simulink library "GFo_Lib"  (R2020b)
settings: Solver=VariableStepAuto  StartTime=0.0  StopTime=10.0  RelTol=1e-3
values from neighbouring files (symbols this model uses):
  Cb = 1/(Zb*wb)    [Init_Base_SM.m]
  fb = fn    [Init_Base_SM.m]
  Ib1 = Sb / (3*Vb1)    [Init_Base_SM.m]
  Ib2 = Sb / (3*Vb2)    [Init_Base_SM.m]
  Lb = Zb/wb    [Init_Base_SM.m]
  Sb = Pb/cos_phi_n    [Init_Base_SM.m]
  Va0 = Vvsc0*sqrt(2)*Vb1*sin(Theta_vsc0*pi/180)    [Init_LF_L_mod.m]
  Vb0 = Vvsc0*sqrt(2)*Vb1*sin(Theta_vsc0*pi/180-2*pi/3)    [Init_LF_L_mod.m]
  Vb1 = Vn1    [Init_Base_SM.m]
  Vb2 = Vn2    [Init_Base_SM.m]
  Vc0 = Vvsc0*sqrt(2)*Vb1*sin(Theta_vsc0*pi/180+2*pi/3)    [Init_LF_L_mod.m]
  Vvsc0 = abs(V1)    [Init_LF_L_mod.m]    (also in Init_LF_SM.m = Vm0)
  Zb = (3*Vb1^2)/Sb    [Init_Base_SM.m]
undefined symbols (not defined in the file or in its folder): C_line, DiscIntNeverNeededParam, Eg0, Is0_d, Is0_q, Kp_Rvi_pu, Time_Step, Ug, VSC01_id0
libraries: powerlib x152, Control_Lib x35, powerlib_meascontrol x10, simulink x6
(part 5 of 5)

== system GFo_Lib/MMC_GFM_EB/Bridge_Model/MMC Average Model/Arm_la ==
  m : Inport
  Controlled Current Source : powerlib/Electrical Sources/Controlled Current Source  Initialize=on  Source_Type=DC  Amplitude=0  Phase=0  Frequency=0  Measurements=None
  Controlled Voltage Source2 : powerlib/Electrical Sources/Controlled Voltage Source  Initialize=on  Source_Type=DC  Amplitude=Vdc/2  Phase=180  Frequency=0  Measurements=None
  Current Measurement7 : powerlib/Measurements/Current Measurement  PhasorSimulation=off  OutputType=Complex  PSBequivalent=0
  Memory1 : Memory  InitialCondition=Vdc/2
  Memory2 : Memory
  Product : Product  RndMeth=Zero
  Product1 : Product  RndMeth=Zero
  Series RLC Branch : powerlib/Elements/Series RLC Branch  LConnTagsString=__new0  RConnTagsString=__new0  BranchType=C  Resistance=1  Inductance=1e-3  SetiL0=off  InitialCurrent=0  Capacitance=C_arm  Setx0=on  InitialVoltage=Vdc  Measurements=None
  Voltage Measurement : powerlib/Measurements/Voltage Measurement  PhasorSimulation=off  OutputType=Complex  PSBequivalent=0
  Voltage Measurement1 : powerlib/Measurements/Voltage Measurement  PhasorSimulation=off  OutputType=Complex  PSBequivalent=0
  V+ : PMIOPort  Side=Left
  V- : PMIOPort  Port=2  Side=Left
  vctot : Outport
  i_arm : Outport  Port=2
  v_arm : Outport  Port=3
  wires:
  Memory1/1 -> Controlled Voltage Source2/1
  Memory2/1 -> Controlled Current Source/1
  Product/1 -> Memory1/1
  Voltage Measurement/1 -> v_arm/1
  Product1/1 -> Memory2/1
  m/1 -> [m], Product1/1
  Current Measurement7/1 -> i_arm/1, Product1/2
  [m] -> Product/2
  Voltage Measurement1/1 -> Product/1, vctot/1
  connections:
  Current Measurement7/RConn1 -- Controlled Voltage Source2/RConn1
  Current Measurement7/LConn1 -- Voltage Measurement/LConn1 -- V+/RConn1
  Controlled Current Source/LConn1 -- Series RLC Branch/RConn1 -- Voltage Measurement1/LConn2 -- V-/RConn1 -- Voltage Measurement/LConn2 -- Controlled Voltage Source2/LConn1
  Controlled Current Source/RConn1 -- Series RLC Branch/LConn1 -- Voltage Measurement1/LConn1

== system GFo_Lib/MMC_GFM_EB/Bridge_Model/MMC Average Model/Arm_lb ==
  m : Inport
  Controlled Current Source : powerlib/Electrical Sources/Controlled Current Source  Initialize=on  Source_Type=DC  Amplitude=0  Phase=0  Frequency=0  Measurements=None
  Controlled Voltage Source2 : powerlib/Electrical Sources/Controlled Voltage Source  Initialize=on  Source_Type=DC  Amplitude=Vdc/2  Phase=180  Frequency=0  Measurements=None
  Current Measurement7 : powerlib/Measurements/Current Measurement  PhasorSimulation=off  OutputType=Complex  PSBequivalent=0
  Memory1 : Memory  InitialCondition=Vdc/2
  Memory2 : Memory
  Product : Product  RndMeth=Zero
  Product1 : Product  RndMeth=Zero
  Series RLC Branch : powerlib/Elements/Series RLC Branch  LConnTagsString=__new0  RConnTagsString=__new0  BranchType=C  Resistance=1  Inductance=1e-3  SetiL0=off  InitialCurrent=0  Capacitance=C_arm  Setx0=on  InitialVoltage=Vdc  Measurements=None
  Voltage Measurement : powerlib/Measurements/Voltage Measurement  PhasorSimulation=off  OutputType=Complex  PSBequivalent=0
  Voltage Measurement1 : powerlib/Measurements/Voltage Measurement  PhasorSimulation=off  OutputType=Complex  PSBequivalent=0
  V+ : PMIOPort  Side=Left
  V- : PMIOPort  Port=2  Side=Left
  vctot : Outport
  i_arm : Outport  Port=2
  v_arm : Outport  Port=3
  wires:
  Memory1/1 -> Controlled Voltage Source2/1
  Memory2/1 -> Controlled Current Source/1
  Product/1 -> Memory1/1
  Voltage Measurement/1 -> v_arm/1
  Product1/1 -> Memory2/1
  m/1 -> [m], Product1/1
  Current Measurement7/1 -> i_arm/1, Product1/2
  [m] -> Product/2
  Voltage Measurement1/1 -> Product/1, vctot/1
  connections:
  Current Measurement7/RConn1 -- Controlled Voltage Source2/RConn1
  Current Measurement7/LConn1 -- Voltage Measurement/LConn1 -- V+/RConn1
  Controlled Current Source/LConn1 -- Series RLC Branch/RConn1 -- Voltage Measurement1/LConn2 -- V-/RConn1 -- Voltage Measurement/LConn2 -- Controlled Voltage Source2/LConn1
  Controlled Current Source/RConn1 -- Series RLC Branch/LConn1 -- Voltage Measurement1/LConn1

== system GFo_Lib/MMC_GFM_EB/Bridge_Model/MMC Average Model/Arm_lc ==
  m : Inport
  Controlled Current Source : powerlib/Electrical Sources/Controlled Current Source  Initialize=on  Source_Type=DC  Amplitude=0  Phase=0  Frequency=0  Measurements=None
  Controlled Voltage Source2 : powerlib/Electrical Sources/Controlled Voltage Source  Initialize=on  Source_Type=DC  Amplitude=Vdc/2  Phase=180  Frequency=0  Measurements=None
  Current Measurement7 : powerlib/Measurements/Current Measurement  PhasorSimulation=off  OutputType=Complex  PSBequivalent=0
  Memory1 : Memory  InitialCondition=Vdc/2
  Memory2 : Memory
  Product : Product  RndMeth=Zero
  Product1 : Product  RndMeth=Zero
  Series RLC Branch : powerlib/Elements/Series RLC Branch  LConnTagsString=__new0  RConnTagsString=__new0  BranchType=C  Resistance=1  Inductance=1e-3  SetiL0=off  InitialCurrent=0  Capacitance=C_arm  Setx0=on  InitialVoltage=Vdc  Measurements=None
  Voltage Measurement : powerlib/Measurements/Voltage Measurement  PhasorSimulation=off  OutputType=Complex  PSBequivalent=0
  Voltage Measurement1 : powerlib/Measurements/Voltage Measurement  PhasorSimulation=off  OutputType=Complex  PSBequivalent=0
  V+ : PMIOPort  Side=Left
  V- : PMIOPort  Port=2  Side=Left
  vctot : Outport
  i_arm : Outport  Port=2
  v_arm : Outport  Port=3
  wires:
  Memory1/1 -> Controlled Voltage Source2/1
  Memory2/1 -> Controlled Current Source/1
  Product/1 -> Memory1/1
  Voltage Measurement/1 -> v_arm/1
  Product1/1 -> Memory2/1
  m/1 -> [m], Product1/1
  Current Measurement7/1 -> i_arm/1, Product1/2
  [m] -> Product/2
  Voltage Measurement1/1 -> Product/1, vctot/1
  connections:
  Current Measurement7/RConn1 -- Controlled Voltage Source2/RConn1
  Current Measurement7/LConn1 -- Voltage Measurement/LConn1 -- V+/RConn1
  Controlled Current Source/LConn1 -- Series RLC Branch/RConn1 -- Voltage Measurement1/LConn2 -- V-/RConn1 -- Voltage Measurement/LConn2 -- Controlled Voltage Source2/LConn1
  Controlled Current Source/RConn1 -- Series RLC Branch/LConn1 -- Voltage Measurement1/LConn1

== system GFo_Lib/MMC_GFM_EB/Bridge_Model/MMC Average Model/Arm_ua ==
  m : Inport
  Controlled Current Source : powerlib/Electrical Sources/Controlled Current Source  Initialize=on  Source_Type=DC  Amplitude=0  Phase=0  Frequency=0  Measurements=None
  Controlled Voltage Source2 : powerlib/Electrical Sources/Controlled Voltage Source  Initialize=on  Source_Type=DC  Amplitude=Vdc/2  Phase=180  Frequency=0  Measurements=None
  Current Measurement7 : powerlib/Measurements/Current Measurement  PhasorSimulation=off  OutputType=Complex  PSBequivalent=0
  Memory1 : Memory  InitialCondition=Vdc/2
  Memory2 : Memory
  Product : Product  RndMeth=Zero
  Product1 : Product  RndMeth=Zero
  Series RLC Branch : powerlib/Elements/Series RLC Branch  LConnTagsString=__new0  RConnTagsString=__new0  BranchType=C  Resistance=1  Inductance=1e-3  SetiL0=off  InitialCurrent=0  Capacitance=C_arm  Setx0=on  InitialVoltage=Vdc  Measurements=None
  Voltage Measurement : powerlib/Measurements/Voltage Measurement  PhasorSimulation=off  OutputType=Complex  PSBequivalent=0
  Voltage Measurement1 : powerlib/Measurements/Voltage Measurement  PhasorSimulation=off  OutputType=Complex  PSBequivalent=0
  V+ : PMIOPort  Side=Left
  V- : PMIOPort  Port=2  Side=Left
  vctot : Outport
  i_arm : Outport  Port=2
  v_arm : Outport  Port=3
  wires:
  Memory1/1 -> Controlled Voltage Source2/1
  Memory2/1 -> Controlled Current Source/1
  Product/1 -> Memory1/1
  Voltage Measurement/1 -> v_arm/1
  Product1/1 -> Memory2/1
  m/1 -> [m], Product1/1
  Current Measurement7/1 -> i_arm/1, Product1/2
  [m] -> Product/2
  Voltage Measurement1/1 -> Product/1, vctot/1
  connections:
  Current Measurement7/RConn1 -- Controlled Voltage Source2/RConn1
  Current Measurement7/LConn1 -- Voltage Measurement/LConn1 -- V+/RConn1
  Controlled Current Source/LConn1 -- Series RLC Branch/RConn1 -- Voltage Measurement1/LConn2 -- V-/RConn1 -- Voltage Measurement/LConn2 -- Controlled Voltage Source2/LConn1
  Controlled Current Source/RConn1 -- Series RLC Branch/LConn1 -- Voltage Measurement1/LConn1

== system GFo_Lib/MMC_GFM_EB/Bridge_Model/MMC Average Model/Arm_ub ==
  m : Inport
  Controlled Current Source : powerlib/Electrical Sources/Controlled Current Source  Initialize=on  Source_Type=DC  Amplitude=0  Phase=0  Frequency=0  Measurements=None
  Controlled Voltage Source2 : powerlib/Electrical Sources/Controlled Voltage Source  Initialize=on  Source_Type=DC  Amplitude=Vdc/2  Phase=180  Frequency=0  Measurements=None
  Current Measurement7 : powerlib/Measurements/Current Measurement  PhasorSimulation=off  OutputType=Complex  PSBequivalent=0
  Memory1 : Memory  InitialCondition=Vdc/2
  Memory2 : Memory
  Product : Product  RndMeth=Zero
  Product1 : Product  RndMeth=Zero
  Series RLC Branch : powerlib/Elements/Series RLC Branch  LConnTagsString=__new0  RConnTagsString=__new0  BranchType=C  Resistance=1  Inductance=1e-3  SetiL0=off  InitialCurrent=0  Capacitance=C_arm  Setx0=on  InitialVoltage=Vdc  Measurements=None
  Voltage Measurement : powerlib/Measurements/Voltage Measurement  PhasorSimulation=off  OutputType=Complex  PSBequivalent=0
  Voltage Measurement1 : powerlib/Measurements/Voltage Measurement  PhasorSimulation=off  OutputType=Complex  PSBequivalent=0
  V+ : PMIOPort  Side=Left
  V- : PMIOPort  Port=2  Side=Left
  vctot : Outport
  i_arm : Outport  Port=2
  v_arm : Outport  Port=3
  wires:
  Memory1/1 -> Controlled Voltage Source2/1
  Memory2/1 -> Controlled Current Source/1
  Product/1 -> Memory1/1
  Voltage Measurement/1 -> v_arm/1
  Product1/1 -> Memory2/1
  m/1 -> [m], Product1/1
  Current Measurement7/1 -> i_arm/1, Product1/2
  [m] -> Product/2
  Voltage Measurement1/1 -> Product/1, vctot/1
  connections:
  Current Measurement7/RConn1 -- Controlled Voltage Source2/RConn1
  Current Measurement7/LConn1 -- Voltage Measurement/LConn1 -- V+/RConn1
  Controlled Current Source/LConn1 -- Series RLC Branch/RConn1 -- Voltage Measurement1/LConn2 -- V-/RConn1 -- Voltage Measurement/LConn2 -- Controlled Voltage Source2/LConn1
  Controlled Current Source/RConn1 -- Series RLC Branch/LConn1 -- Voltage Measurement1/LConn1

== system GFo_Lib/MMC_GFM_EB/Bridge_Model/MMC Average Model/Arm_uc ==
  m : Inport
  Controlled Current Source : powerlib/Electrical Sources/Controlled Current Source  Initialize=on  Source_Type=DC  Amplitude=0  Phase=0  Frequency=0  Measurements=None
  Controlled Voltage Source2 : powerlib/Electrical Sources/Controlled Voltage Source  Initialize=on  Source_Type=DC  Amplitude=Vdc/2  Phase=180  Frequency=0  Measurements=None
  Current Measurement7 : powerlib/Measurements/Current Measurement  PhasorSimulation=off  OutputType=Complex  PSBequivalent=0
  Memory1 : Memory  InitialCondition=Vdc/2
  Memory2 : Memory
  Product : Product  RndMeth=Zero
  Product1 : Product  RndMeth=Zero
  Series RLC Branch : powerlib/Elements/Series RLC Branch  LConnTagsString=__new0  RConnTagsString=__new0  BranchType=C  Resistance=1  Inductance=1e-3  SetiL0=off  InitialCurrent=0  Capacitance=C_arm  Setx0=on  InitialVoltage=Vdc  Measurements=None
  Voltage Measurement : powerlib/Measurements/Voltage Measurement  PhasorSimulation=off  OutputType=Complex  PSBequivalent=0
  Voltage Measurement1 : powerlib/Measurements/Voltage Measurement  PhasorSimulation=off  OutputType=Complex  PSBequivalent=0
  V+ : PMIOPort  Side=Left
  V- : PMIOPort  Port=2  Side=Left
  vctot : Outport
  i_arm : Outport  Port=2
  v_arm : Outport  Port=3
  wires:
  Memory1/1 -> Controlled Voltage Source2/1
  Memory2/1 -> Controlled Current Source/1
  Product/1 -> Memory1/1
  Voltage Measurement/1 -> v_arm/1
  Product1/1 -> Memory2/1
  m/1 -> [m], Product1/1
  Current Measurement7/1 -> i_arm/1, Product1/2
  [m] -> Product/2
  Voltage Measurement1/1 -> Product/1, vctot/1
  connections:
  Current Measurement7/RConn1 -- Controlled Voltage Source2/RConn1
  Current Measurement7/LConn1 -- Voltage Measurement/LConn1 -- V+/RConn1
  Controlled Current Source/LConn1 -- Series RLC Branch/RConn1 -- Voltage Measurement1/LConn2 -- V-/RConn1 -- Voltage Measurement/LConn2 -- Controlled Voltage Source2/LConn1
  Controlled Current Source/RConn1 -- Series RLC Branch/LConn1 -- Voltage Measurement1/LConn1

== system GFo_Lib/MMC_GFM_EB/Control loops/Current Limitation/Current control ==
  Ig_dq0* : Inport
  Ig_dq0 : Inport  Port=2
  vg_dq0 : Inport  Port=3
  w : Inport  Port=4
  Demux : Demux  Outputs=2
  Demux1 : Demux  Outputs=2
  Demux2 : Demux  Outputs=2
  Gain Corrector : Gain  Gain=3/(Tr_I_max/1000)*Lt_pu
  Gain Corrector1 : Gain  Gain=3/(Tr_I_max/1000)*Lt_pu
  Mux : Mux  Inputs=2
  Product : Product  RndMeth=Zero
  Product1 : Product  RndMeth=Zero
  Sum : Sum  Inputs=|+-
  Sum2 : Sum  Inputs=|+-
  Sum3 : Sum  Inputs=|++
  Sum5 : Sum  Inputs=++|
  Sum6 : Sum  Inputs=-+|
  Sum7 : Sum  Inputs=++|
  vpcc_abc{1,3..6} (5 alike) : Scope
  w*Lf_pu : Gain  Gain=Lt_pu
  vm : Outport  InitialOutput=0  VectorParamsAs1DForOutWhenUnconnected=off
  wires:
  Demux2/2 -> Sum7/1
  Demux2/1 -> Sum3/2
  w/1 -> vpcc_abc5/1, w*Lf_pu/1
  Sum/1 -> vpcc_abc1/1, Gain Corrector/1
  Sum7/1 -> Mux/2  "Vm_q*"
  Sum3/1 -> Mux/1, vpcc_abc3/1  "Vm_d*"
  Sum5/1 -> Sum7/2
  Product1/1 -> Sum5/1
  Gain Corrector1/1 -> Sum5/2
  Demux/2 -> Sum6/2
  Sum2/1 -> Sum3/1
  Product/1 -> Sum2/2
  Demux1/2 -> Sum6/1, Product/1
  w*Lf_pu/1 -> Product/2, Product1/1
  Gain Corrector/1 -> Sum2/1
  Demux1/1 -> Sum/2, Product1/2
  Demux/1 -> Sum/1
  Ig_dq0/1 -> Demux1/1
  vg_dq0/1 -> Demux2/1, vpcc_abc6/1
  Sum6/1 -> Gain Corrector1/1
  Ig_dq0*/1 -> vpcc_abc4/1, Demux/1
  Mux/1 -> vm/1

== system GFo_Lib/MMC_GFM_EB/Control loops/Current Limitation/Inverse Current control ==
  Vm_dq* : Inport
  Ig_dq : Inport  Port=2
  vg_dq : Inport  Port=3
  w : Inport  Port=4
  Demux : Demux  Outputs=2
  Demux1 : Demux  Outputs=2
  Demux2 : Demux  Outputs=2
  Gain Corrector2 : Gain  Gain=1/(3/(Tr_I_max/1000)*Lt_pu)
  Gain Corrector3 : Gain  Gain=1/(3/(Tr_I_max/1000)*Lt_pu)
  Mux : Mux  Inputs=2
  Product : Product  RndMeth=Zero
  Product1 : Product  RndMeth=Zero
  Sum : Sum  Inputs=|+-
  Sum2 : Sum  Inputs=|++
  Sum3 : Sum  Inputs=|++
  Sum5 : Sum  Inputs=-+|
  Sum6 : Sum  Inputs=-+|
  Sum7 : Sum  Inputs=++|
  w*Lf_pu : Gain  Gain=Lt_pu
  Is_dq* : Outport  InitialOutput=0  VectorParamsAs1DForOutWhenUnconnected=off
  wires:
  vg_dq/1 -> Demux2/1
  Ig_dq/1 -> Demux1/1
  Vm_dq*/1 -> Demux/1
  Demux/1 -> Sum/1
  Demux1/1 -> Sum3/2, Product1/2
  Sum/1 -> Sum2/1
  w*Lf_pu/1 -> Product1/1, Product/2
  Product/1 -> Sum2/2
  Sum2/1 -> Gain Corrector3/1
  Mux/1 -> Is_dq*/1
  Demux/2 -> Sum6/2
  Sum6/1 -> Sum5/2
  Sum5/1 -> Gain Corrector2/1
  Sum3/1 -> Mux/1  "is_d*"
  Sum7/1 -> Mux/2  "is_q*"
  w/1 -> w*Lf_pu/1
  Demux1/2 -> Sum7/1, Product/1
  Gain Corrector3/1 -> Sum3/1
  Demux2/1 -> Sum/2
  Demux2/2 -> Sum6/1
  Product1/1 -> Sum5/1
  Gain Corrector2/1 -> Sum7/2

== system GFo_Lib/MMC_GFM_EB/Control loops/DC part: stored energy control + differential current control/Control Wdiff ==
  Wdiff pu : Inport
  Wdiff_ref pu : Inport  Port=2
  theta : Inport  Port=3
  vv_pu : Inport  Port=4
  Constant : Constant  Value=-2
  Discrete-Time Integrator : DiscreteIntegrator  SampleTime=Time_Step  ICPrevOutput=DiscIntNeverNeededParam  ICPrevScaledInput=DiscIntNeverNeededParam
  Gain5 : Gain  Gain=Vb1/Vdcb
  Gain_i 1 : Gain  Gain=Ki_Wdiff_pu  SaturateOnIntegerOverflow=on  OutDataTypeStr=Inherit: Same as input  ParamDataTypeStr=Inherit: Same as input
  Gain_i 4 : Gain  Gain=Kp_Wdiff_pu  SaturateOnIntegerOverflow=on  OutDataTypeStr=Inherit: Same as input  ParamDataTypeStr=Inherit: Same as input
  Mux1 : Mux  Inputs=3
  Mux2 : Mux  Inputs=3
  Mux3 : Mux  Inputs=3
  Mux5 : Mux  Inputs=2
  Product1 : Product  Inputs=*/*
  Sum2 : Sum  InputSameDT=on  SaturateOnIntegerOverflow=on  OutDataTypeStr=Inherit: Same as first input
  Sum3 : Sum  Inputs=+-  InputSameDT=on  SaturateOnIntegerOverflow=on  OutDataTypeStr=Inherit: Same as first input
  vsa_1 : Fcn  Expr=u(1)*cos(u(4))
  vsa_2 : Fcn  Expr=u(1)-1/2*u(2)-1/2*u(3)
  vsa_3 : Fcn  Expr=u(1)*cos(u(4))+1/3^0.5*u(2)*cos(u(4)+1/2*pi)+1/3^0.5*u(3)*cos(u(4)-1/2*pi)
  vsb_1 : Fcn  Expr=-1/2*u(1)+u(2)-1/2*u(3)
  vsb_2 : Fcn  Expr=u(2)*cos(u(4)-2/3*pi)
  vsb_3 : Fcn  Expr=u(3)*cos(u(4)+2/3*pi)
  vsb_4 : Fcn  Expr=-1/2*u(1)-1/2*u(2)+u(3)
  vsb_5 : Fcn  Expr=1/3^0.5*u(1)*cos(u(4)-7/6*pi)+u(2)*cos(u(4)-2/3*pi)+1/3^0.5*u(3)*cos(u(4)-1/6*pi)
  vsb_6 : Fcn  Expr=1/3^0.5*u(1)*cos(u(4)+7/6*pi)+1/3^0.5*u(2)*cos(u(4)+1/6*pi)+u(3)*cos(u(4)+2/3*pi)
  Idiff ref pu : Outport
  Idiff ref pu1 : Outport  Port=2
  wires:
  Wdiff pu/1 -> Sum3/2
  Wdiff_ref pu/1 -> Sum3/1
  vsb_2/1 -> Mux1/2
  vsa_1/1 -> Mux1/1
  vsb_3/1 -> Mux1/3
  Product1/1 -> Mux5/1  "Idiff_ac_pu"
  vsa_2/1 -> Mux2/1
  vsb_1/1 -> Mux2/2
  vsb_4/1 -> Mux2/3
  vsb_6/1 -> Mux3/3
  vsa_3/1 -> Mux3/1
  vsb_5/1 -> Mux3/2
  Mux5/1 -> vsa_3/1, vsb_5/1, vsb_6/1, vsa_1/1, vsb_2/1, vsb_3/1
  theta/1 -> Mux5/2
  Mux3/1 -> Idiff ref pu/1
  Discrete-Time Integrator/1 -> Sum2/1
  Gain5/1 -> Product1/3
  Gain_i 1/1 -> Discrete-Time Integrator/1
  vv_pu/1 -> Gain5/1
  Sum3/1 -> Gain_i 4/1, Gain_i 1/1
  Sum2/1 -> Product1/1
  Gain_i 4/1 -> Sum2/2
  Mux1/1 -> vsa_2/1, vsb_4/1, vsb_1/1
  Mux2/1 -> Idiff ref pu1/1
  Constant/1 -> Product1/2

== system GFo_Lib/MMC_GFM_EB/Control loops/DC part: stored energy control + differential current control/Control Wtot  ==
  note: Reference of i_diff --> adjusting dc power
  note: Energy based control
      |
      | dW
      | ----- = Pdc - Pac --> In this simulation, the energy is regulated by adjusting dc power
      | dt
      |
      | Pdc = PIcontroller*(W_ref - W_mes) + Pac
  note: ac power is considered as a disturbance
  Wtot_pu : Inport
  Wtot ref pu : Inport  Port=2
  p_ac_pu : Inport  Port=3
  Vdc_pu : Inport  Port=4
  Discrete-Time Integrator : DiscreteIntegrator  SampleTime=Time_Step  ICPrevOutput=DiscIntNeverNeededParam  ICPrevScaledInput=DiscIntNeverNeededParam
  Divide1 : Product  Inputs=/*
  Gain1 : Gain  Gain=1/3
  Gain_i 1 : Gain  Gain=Kp_Wtot_pu  SaturateOnIntegerOverflow=on  OutDataTypeStr=Inherit: Same as input  ParamDataTypeStr=Inherit: Same as input
  Gain_i 5 : Gain  Gain=Ki_Wtot_pu  SaturateOnIntegerOverflow=on  OutDataTypeStr=Inherit: Same as input  ParamDataTypeStr=Inherit: Same as input
  Scope{1..4} (4 alike) : Scope
      settings: Tag=op_tm_save_it
  Sum : Sum  Inputs=++|
  Sum1 : Sum  InputSameDT=on  SaturateOnIntegerOverflow=on  OutDataTypeStr=Inherit: Same as first input
  Sum4 : Sum  Inputs=+-  InputSameDT=on  SaturateOnIntegerOverflow=on  OutDataTypeStr=Inherit: Same as first input
  Idiff ref pu : Outport
  wires:
  Sum/1 -> Scope3/1, Divide1/2
  Divide1/1 -> Scope1/1, Idiff ref pu/1  "idiff_ref"
  Vdc_pu/1 -> Divide1/1
  Sum1/1 -> Scope2/1, Sum/2
  Sum4/1 -> Scope4/1, Gain_i 1/1, Gain_i 5/1
  Gain_i 5/1 -> Discrete-Time Integrator/1
  Discrete-Time Integrator/1 -> Sum1/1
  Gain_i 1/1 -> Sum1/2
  Wtot ref pu/1 -> Sum4/1
  Wtot_pu/1 -> Sum4/2
  p_ac_pu/1 -> Gain1/1
  Gain1/1 -> Sum/1

== system GFo_Lib/MMC_GFM_EB/Control loops/DC part: stored energy control + differential current control/Differential_current_control ==
  vdc_pu : Inport
  idiff_pu : Inport  Port=2
  idiff_ref_pu : Inport  Port=3
  Discrete-Time Integrator : DiscreteIntegrator  SampleTime=Time_Step  ICPrevOutput=DiscIntNeverNeededParam  ICPrevScaledInput=DiscIntNeverNeededParam
  Gain3 : Gain  Gain=1/2
  Gain_i 1 : Gain  Gain=Diff_CC_kp  SaturateOnIntegerOverflow=on  OutDataTypeStr=Inherit: Same as input  ParamDataTypeStr=Inherit: Same as input
  Gain_i 5 : Gain  Gain=Diff_CC_ki  SaturateOnIntegerOverflow=on  OutDataTypeStr=Inherit: Same as input  ParamDataTypeStr=Inherit: Same as input
  Sum1 : Sum  Inputs=+-  InputSameDT=on  SaturateOnIntegerOverflow=on  OutDataTypeStr=Inherit: Same as first input
  Sum2 : Sum  InputSameDT=on  SaturateOnIntegerOverflow=on  OutDataTypeStr=Inherit: Same as first input
  Sum3 : Sum  Inputs=+-  InputSameDT=on  SaturateOnIntegerOverflow=on  OutDataTypeStr=Inherit: Same as first input
  Vprediff_ref_pu : Outport
  wires:
  idiff_pu/1 -> Sum1/2
  idiff_ref_pu/1 -> Sum1/1
  Sum1/1 -> Gain_i 1/1, Gain_i 5/1
  Gain_i 5/1 -> Discrete-Time Integrator/1
  Gain_i 1/1 -> Sum2/2
  Discrete-Time Integrator/1 -> Sum2/1
  vdc_pu/1 -> Gain3/1
  Gain3/1 -> Sum3/1
  Sum3/1 -> Vprediff_ref_pu/1
  Sum2/1 -> Sum3/2

== system GFo_Lib/MMC_GFM_EB/Control loops/DC part: stored energy control + differential current control/Wdiff computation ==
  vctot u_pu : Inport
  vctot l_pu : Inport  Port=2
  Gain10 : Gain  Gain=1/2
  Product : Product
  Product1 : Product
  Second-Order Filter : powerlib_meascontrol/Filters/Second-Order Filter  FilterType=Bandstop (Notch)  Fo=fb  Zeta=1  Ts=0  Initialize=on  Vac_Init="[0,  0,  60; 0, 0, 60; 0, 0, 60]"  Vdc_Init=[0, 0, 0]  PlotResponse=off  FreqRange=[0, 500, 1]
      settings: SourceProductBaseCode=PS
  Sum3 : Sum  Inputs=+-
  Wdiff : Outport  PortDimensions=3
  wires:
  vctot u_pu/1 -> Product/2, Product/1
  Sum3/1 -> Gain10/1
  vctot l_pu/1 -> Product1/2, Product1/1
  Product/1 -> Sum3/1
  Product1/1 -> Sum3/2
  Second-Order Filter/1 -> Wdiff/1
  Gain10/1 -> Second-Order Filter/1

== system GFo_Lib/MMC_GFM_EB/Control loops/DC part: stored energy control + differential current control/Wtot computation ==
  vctot u_pu : Inport
  vctot l_pu : Inport  Port=2
  Gain10 : Gain  Gain=1/2
  Product : Product
  Product1 : Product
  Second-Order Filter : powerlib_meascontrol/Filters/Second-Order Filter  FilterType=Bandstop (Notch)  Fo=2*fb  Zeta=1  Ts=0  Initialize=on  Vac_Init="[0,  0,  60; 0, 0, 60; 0, 0, 60]"  Vdc_Init=[1; 1; 1]  PlotResponse=off  FreqRange=[0, 500, 1]
      settings: SourceProductBaseCode=PS
  Sum3 : Sum
  Wtot : Outport  PortDimensions=3
  wires:
  vctot u_pu/1 -> Product/2, Product/1
  Sum3/1 -> Gain10/1
  vctot l_pu/1 -> Product1/2, Product1/1
  Product/1 -> Sum3/1
  Product1/1 -> Sum3/2
  Second-Order Filter/1 -> Wtot/1
  Gain10/1 -> Second-Order Filter/1

== system GFo_Lib/MMC_GFM_EB/Control loops/Transient Damping Resistance/Filter w_LF ==
  e : Inport
  1/T_LP : Gain  Gain=W_TVR  SaturateOnIntegerOverflow=on  OutDataTypeStr=Inherit: Same as input  ParamDataTypeStr=Inherit: Same as input
  Integrator : Integrator  InitialConditionSource=external  InitialCondition=[VSC01_id0*0.04]
  Sum1 : Sum  Inputs=|+-  InputSameDT=on  SaturateOnIntegerOverflow=on  OutDataTypeStr=Inherit: Same as first input
  s : Outport  VectorParamsAs1DForOutWhenUnconnected=off
  wires:
  e/1 -> Sum1/1, Integrator/2
  Integrator/1 -> s/1, Sum1/2
  1/T_LP/1 -> Integrator/1
  Sum1/1 -> 1/T_LP/1

== system GFo_Lib/MMC_GFM_EB/Control loops/VI/dq to phasor ==
  dq_mes : Inport
  Demux : Demux  Outputs=2
      settings: DisplayOption=none
  Sqrt : Sqrt  SaturateOnIntegerOverflow=on
  Sum4 : Sum  Inputs=|++  InputSameDT=on  SaturateOnIntegerOverflow=on  OutDataTypeStr=Inherit: Same as first input
  Vrdird : Product  InputSameDT=on  RndMeth=Zero  SaturateOnIntegerOverflow=on  OutDataTypeStr=Inherit: Same as first input
  Vrqirq : Product  InputSameDT=on  RndMeth=Zero  SaturateOnIntegerOverflow=on  OutDataTypeStr=Inherit: Same as first input
  rms : Outport  VectorParamsAs1DForOutWhenUnconnected=off
  wires:
  Sum4/1 -> Sqrt/1
  Vrqirq/1 -> Sum4/2
  Vrdird/1 -> Sum4/1
  Demux/2 -> Vrqirq/2, Vrqirq/1
  Demux/1 -> Vrdird/2, Vrdird/1
  dq_mes/1 -> Demux/1
  Sqrt/1 -> rms/1

== system GFo_Lib/Mean Model 2-Level L-filter/Control loops/Current Limitation/Current control ==
  Ig_dq0* : Inport
  Ig_dq0 : Inport  Port=2
  vg_dq0 : Inport  Port=3
  w : Inport  Port=4
  Demux : Demux  Outputs=2
  Demux1 : Demux  Outputs=2
  Demux2 : Demux  Outputs=2
  Gain Corrector : Gain  Gain=3/(Tr_I_max/1000)*Lt_pu
  Gain Corrector1 : Gain  Gain=3/(Tr_I_max/1000)*Lt_pu
  Mux : Mux  Inputs=2
  Product : Product  RndMeth=Zero
  Product1 : Product  RndMeth=Zero
  Sum : Sum  Inputs=|+-
  Sum2 : Sum  Inputs=|+-
  Sum3 : Sum  Inputs=|++
  Sum5 : Sum  Inputs=++|
  Sum6 : Sum  Inputs=-+|
  Sum7 : Sum  Inputs=++|
  vpcc_abc{1,3..6} (5 alike) : Scope
  w*Lf_pu : Gain  Gain=Lt_pu
  vm : Outport  InitialOutput=0  VectorParamsAs1DForOutWhenUnconnected=off
  wires:
  Mux/1 -> vm/1
  Ig_dq0*/1 -> Demux/1, vpcc_abc4/1
  Sum6/1 -> Gain Corrector1/1
  vg_dq0/1 -> vpcc_abc6/1, Demux2/1
  Ig_dq0/1 -> Demux1/1
  Demux/1 -> Sum/1
  Demux1/1 -> Product1/2, Sum/2
  Gain Corrector/1 -> Sum2/1
  w*Lf_pu/1 -> Product1/1, Product/2
  Demux1/2 -> Product/1, Sum6/1
  Product/1 -> Sum2/2
  Sum2/1 -> Sum3/1
  Demux/2 -> Sum6/2
  Gain Corrector1/1 -> Sum5/2
  Product1/1 -> Sum5/1
  Sum5/1 -> Sum7/2
  Sum3/1 -> vpcc_abc3/1, Mux/1  "Vm_d*"
  Sum7/1 -> Mux/2  "Vm_q*"
  Sum/1 -> Gain Corrector/1, vpcc_abc1/1
  w/1 -> w*Lf_pu/1, vpcc_abc5/1
  Demux2/1 -> Sum3/2
  Demux2/2 -> Sum7/1

== system GFo_Lib/Mean Model 2-Level L-filter/Control loops/Current Limitation/Inverse Current control ==
  Vm_dq* : Inport
  Ig_dq : Inport  Port=2
  vg_dq : Inport  Port=3
  w : Inport  Port=4
  Demux : Demux  Outputs=2
  Demux1 : Demux  Outputs=2
  Demux2 : Demux  Outputs=2
  Gain Corrector2 : Gain  Gain=1/(3/(Tr_I_max/1000)*Lt_pu)
  Gain Corrector3 : Gain  Gain=1/(3/(Tr_I_max/1000)*Lt_pu)
  Mux : Mux  Inputs=2
  Product : Product  RndMeth=Zero
  Product1 : Product  RndMeth=Zero
  Sum : Sum  Inputs=|+-
  Sum2 : Sum  Inputs=|++
  Sum3 : Sum  Inputs=|++
  Sum5 : Sum  Inputs=-+|
  Sum6 : Sum  Inputs=-+|
  Sum7 : Sum  Inputs=++|
  w*Lf_pu : Gain  Gain=Lt_pu
  Is_dq* : Outport  InitialOutput=0  VectorParamsAs1DForOutWhenUnconnected=off
  wires:
  Gain Corrector2/1 -> Sum7/2
  Product1/1 -> Sum5/1
  Demux2/2 -> Sum6/1
  Demux2/1 -> Sum/2
  Gain Corrector3/1 -> Sum3/1
  Demux1/2 -> Product/1, Sum7/1
  w/1 -> w*Lf_pu/1
  Sum7/1 -> Mux/2  "is_q*"
  Sum3/1 -> Mux/1  "is_d*"
  Sum5/1 -> Gain Corrector2/1
  Sum6/1 -> Sum5/2
  Demux/2 -> Sum6/2
  Mux/1 -> Is_dq*/1
  Sum2/1 -> Gain Corrector3/1
  Product/1 -> Sum2/2
  w*Lf_pu/1 -> Product/2, Product1/1
  Sum/1 -> Sum2/1
  Demux1/1 -> Product1/2, Sum3/2
  Demux/1 -> Sum/1
  Vm_dq*/1 -> Demux/1
  Ig_dq/1 -> Demux1/1
  vg_dq/1 -> Demux2/1

== system GFo_Lib/Mean Model 2-Level L-filter/Control loops/Transient Damping Resistance/Filter w_LF ==
  e : Inport
  1/T_LP : Gain  Gain=W_TVR  SaturateOnIntegerOverflow=on  OutDataTypeStr=Inherit: Same as input  ParamDataTypeStr=Inherit: Same as input
  Integrator : Integrator  InitialConditionSource=external  InitialCondition=[VSC01_id0*0.04]
  Sum1 : Sum  Inputs=|+-  InputSameDT=on  SaturateOnIntegerOverflow=on  OutDataTypeStr=Inherit: Same as first input
  s : Outport  VectorParamsAs1DForOutWhenUnconnected=off
  wires:
  Sum1/1 -> 1/T_LP/1
  1/T_LP/1 -> Integrator/1
  Integrator/1 -> Sum1/2, s/1
  e/1 -> Integrator/2, Sum1/1

== system GFo_Lib/Mean Model 2-Level L-filter/Control loops/VI/dq to phasor ==
  dq_mes : Inport
  Demux : Demux  Outputs=2
      settings: DisplayOption=none
  Sqrt : Sqrt  SaturateOnIntegerOverflow=on
  Sum4 : Sum  Inputs=|++  InputSameDT=on  SaturateOnIntegerOverflow=on  OutDataTypeStr=Inherit: Same as first input
  Vrdird : Product  InputSameDT=on  RndMeth=Zero  SaturateOnIntegerOverflow=on  OutDataTypeStr=Inherit: Same as first input
  Vrqirq : Product  InputSameDT=on  RndMeth=Zero  SaturateOnIntegerOverflow=on  OutDataTypeStr=Inherit: Same as first input
  rms : Outport  VectorParamsAs1DForOutWhenUnconnected=off
  wires:
  Sqrt/1 -> rms/1
  dq_mes/1 -> Demux/1
  Demux/1 -> Vrdird/1, Vrdird/2
  Demux/2 -> Vrqirq/1, Vrqirq/2
  Vrdird/1 -> Sum4/1
  Vrqirq/1 -> Sum4/2
  Sum4/1 -> Sqrt/1

== system GFo_Lib/Mean Model 2-Level L-filter with DC link/Control loops/Current Limitation/Current control ==
  Ig_dq0* : Inport
  Ig_dq0 : Inport  Port=2
  vg_dq0 : Inport  Port=3
  w : Inport  Port=4
  Demux : Demux  Outputs=2
  Demux1 : Demux  Outputs=2
  Demux2 : Demux  Outputs=2
  Gain Corrector : Gain  Gain=3/(Tr_I_max/1000)*Lt_pu
  Gain Corrector1 : Gain  Gain=3/(Tr_I_max/1000)*Lt_pu
  Mux : Mux  Inputs=2
  Product : Product  RndMeth=Zero
  Product1 : Product  RndMeth=Zero
  Sum : Sum  Inputs=|+-
  Sum2 : Sum  Inputs=|+-
  Sum3 : Sum  Inputs=|++
  Sum5 : Sum  Inputs=++|
  Sum6 : Sum  Inputs=-+|
  Sum7 : Sum  Inputs=++|
  vpcc_abc{1,3..6} (5 alike) : Scope
  w*Lf_pu : Gain  Gain=Lt_pu
  vm : Outport  InitialOutput=0  VectorParamsAs1DForOutWhenUnconnected=off
  wires:
  Mux/1 -> vm/1
  Ig_dq0*/1 -> Demux/1, vpcc_abc4/1
  Sum6/1 -> Gain Corrector1/1
  vg_dq0/1 -> vpcc_abc6/1, Demux2/1
  Ig_dq0/1 -> Demux1/1
  Demux/1 -> Sum/1
  Demux1/1 -> Product1/2, Sum/2
  Gain Corrector/1 -> Sum2/1
  w*Lf_pu/1 -> Product1/1, Product/2
  Demux1/2 -> Product/1, Sum6/1
  Product/1 -> Sum2/2
  Sum2/1 -> Sum3/1
  Demux/2 -> Sum6/2
  Gain Corrector1/1 -> Sum5/2
  Product1/1 -> Sum5/1
  Sum5/1 -> Sum7/2
  Sum3/1 -> vpcc_abc3/1, Mux/1  "Vm_d*"
  Sum7/1 -> Mux/2  "Vm_q*"
  Sum/1 -> Gain Corrector/1, vpcc_abc1/1
  w/1 -> w*Lf_pu/1, vpcc_abc5/1
  Demux2/1 -> Sum3/2
  Demux2/2 -> Sum7/1

== system GFo_Lib/Mean Model 2-Level L-filter with DC link/Control loops/Current Limitation/Inverse Current control ==
  Vm_dq* : Inport
  Ig_dq : Inport  Port=2
  vg_dq : Inport  Port=3
  w : Inport  Port=4
  Demux : Demux  Outputs=2
  Demux1 : Demux  Outputs=2
  Demux2 : Demux  Outputs=2
  Gain Corrector2 : Gain  Gain=1/(3/(Tr_I_max/1000)*Lt_pu)
  Gain Corrector3 : Gain  Gain=1/(3/(Tr_I_max/1000)*Lt_pu)
  Mux : Mux  Inputs=2
  Product : Product  RndMeth=Zero
  Product1 : Product  RndMeth=Zero
  Sum : Sum  Inputs=|+-
  Sum2 : Sum  Inputs=|++
  Sum3 : Sum  Inputs=|++
  Sum5 : Sum  Inputs=-+|
  Sum6 : Sum  Inputs=-+|
  Sum7 : Sum  Inputs=++|
  w*Lf_pu : Gain  Gain=Lt_pu
  Is_dq* : Outport  InitialOutput=0  VectorParamsAs1DForOutWhenUnconnected=off
  wires:
  Gain Corrector2/1 -> Sum7/2
  Product1/1 -> Sum5/1
  Demux2/2 -> Sum6/1
  Demux2/1 -> Sum/2
  Gain Corrector3/1 -> Sum3/1
  Demux1/2 -> Product/1, Sum7/1
  w/1 -> w*Lf_pu/1
  Sum7/1 -> Mux/2  "is_q*"
  Sum3/1 -> Mux/1  "is_d*"
  Sum5/1 -> Gain Corrector2/1
  Sum6/1 -> Sum5/2
  Demux/2 -> Sum6/2
  Mux/1 -> Is_dq*/1
  Sum2/1 -> Gain Corrector3/1
  Product/1 -> Sum2/2
  w*Lf_pu/1 -> Product/2, Product1/1
  Sum/1 -> Sum2/1
  Demux1/1 -> Product1/2, Sum3/2
  Demux/1 -> Sum/1
  Vm_dq*/1 -> Demux/1
  Ig_dq/1 -> Demux1/1
  vg_dq/1 -> Demux2/1

== system GFo_Lib/Mean Model 2-Level L-filter with DC link/Control loops/Transient Damping Resistance/Filter w_LF ==
  e : Inport
  1/T_LP : Gain  Gain=W_TVR  SaturateOnIntegerOverflow=on  OutDataTypeStr=Inherit: Same as input  ParamDataTypeStr=Inherit: Same as input
  Integrator : Integrator  InitialConditionSource=external  InitialCondition=[VSC01_id0*0.04]
  Sum1 : Sum  Inputs=|+-  InputSameDT=on  SaturateOnIntegerOverflow=on  OutDataTypeStr=Inherit: Same as first input
  s : Outport  VectorParamsAs1DForOutWhenUnconnected=off
  wires:
  Sum1/1 -> 1/T_LP/1
  1/T_LP/1 -> Integrator/1
  Integrator/1 -> Sum1/2, s/1
  e/1 -> Integrator/2, Sum1/1

== system GFo_Lib/Mean Model 2-Level L-filter with DC link/Control loops/VI/dq to phasor ==
  dq_mes : Inport
  Demux : Demux  Outputs=2
      settings: DisplayOption=none
  Sqrt : Sqrt  SaturateOnIntegerOverflow=on
  Sum4 : Sum  Inputs=|++  InputSameDT=on  SaturateOnIntegerOverflow=on  OutDataTypeStr=Inherit: Same as first input
  Vrdird : Product  InputSameDT=on  RndMeth=Zero  SaturateOnIntegerOverflow=on  OutDataTypeStr=Inherit: Same as first input
  Vrqirq : Product  InputSameDT=on  RndMeth=Zero  SaturateOnIntegerOverflow=on  OutDataTypeStr=Inherit: Same as first input
  rms : Outport  VectorParamsAs1DForOutWhenUnconnected=off
  wires:
  Sqrt/1 -> rms/1
  dq_mes/1 -> Demux/1
  Demux/1 -> Vrdird/1, Vrdird/2
  Demux/2 -> Vrqirq/1, Vrqirq/2
  Vrdird/1 -> Sum4/1
  Vrqirq/1 -> Sum4/2
  Sum4/1 -> Sqrt/1

== system GFo_Lib/ 2-Level LCL-filter with DC Link/Control loops/Inner Cascaded control loops/Current Limitation/Current control ==
  Ig_dq0* : Inport
  Is_dq0 : Inport  Port=2
  vpcc_dq0 : Inport  Port=3
  w : Inport  Port=4
  Demux : Demux  Outputs=2
  Demux1 : Demux  Outputs=2
  Demux2 : Demux  Outputs=2
  Gain Corrector : Gain  Gain=3/(Tr_I_max/1000)*Lf_pu
  Gain Corrector1 : Gain  Gain=3/(Tr_I_max/1000)*Lf_pu
  Mux : Mux  Inputs=2
  Product : Product  RndMeth=Zero
  Product1 : Product  RndMeth=Zero
  Sum : Sum  Inputs=|+-
  Sum2 : Sum  Inputs=|+-
  Sum3 : Sum  Inputs=|++
  Sum5 : Sum  Inputs=++|
  Sum6 : Sum  Inputs=-+|
  Sum7 : Sum  Inputs=++|
  vpcc_abc{1,3..6} (5 alike) : Scope
  w*Lf_pu : Gain  Gain=Lf_pu
  vm : Outport  InitialOutput=0  VectorParamsAs1DForOutWhenUnconnected=off
  wires:
  Mux/1 -> vm/1
  Ig_dq0*/1 -> Demux/1, vpcc_abc4/1
  Sum6/1 -> Gain Corrector1/1
  vpcc_dq0/1 -> vpcc_abc6/1, Demux2/1
  Is_dq0/1 -> Demux1/1
  Demux/1 -> Sum/1
  Demux1/1 -> Product1/2, Sum/2
  Gain Corrector/1 -> Sum2/1
  w*Lf_pu/1 -> Product1/1, Product/2
  Demux1/2 -> Product/1, Sum6/1
  Product/1 -> Sum2/2
  Sum2/1 -> Sum3/1
  Demux/2 -> Sum6/2
  Gain Corrector1/1 -> Sum5/2
  Product1/1 -> Sum5/1
  Sum5/1 -> Sum7/2
  Sum3/1 -> vpcc_abc3/1, Mux/1  "Vm_d*"
  Sum7/1 -> Mux/2  "Vm_q*"
  Sum/1 -> Gain Corrector/1, vpcc_abc1/1
  w/1 -> w*Lf_pu/1, vpcc_abc5/1
  Demux2/1 -> Sum3/2
  Demux2/2 -> Sum7/1

== system GFo_Lib/ 2-Level LCL-filter with DC Link/Control loops/Inner Cascaded control loops/Current Limitation/Inverse Current control ==
  Vm_dq* : Inport
  Is_dq : Inport  Port=2
  Eg_dq : Inport  Port=3
  w : Inport  Port=4
  Demux : Demux  Outputs=2
  Demux1 : Demux  Outputs=2
  Demux2 : Demux  Outputs=2
  Gain Corrector2 : Gain  Gain=1/(3/(Tr_I_max/1000)*Lf_pu)
  Gain Corrector3 : Gain  Gain=1/(3/(Tr_I_max/1000)*Lf_pu)
  Mux : Mux  Inputs=2
  Product : Product  RndMeth=Zero
  Product1 : Product  RndMeth=Zero
  Sum : Sum  Inputs=|+-
  Sum2 : Sum  Inputs=|++
  Sum3 : Sum  Inputs=|++
  Sum5 : Sum  Inputs=-+|
  Sum6 : Sum  Inputs=-+|
  Sum7 : Sum  Inputs=++|
  w*Lf_pu : Gain  Gain=Lf_pu
  Is_dq* : Outport  InitialOutput=0  VectorParamsAs1DForOutWhenUnconnected=off
  wires:
  Gain Corrector2/1 -> Sum7/2
  Product1/1 -> Sum5/1
  Demux2/2 -> Sum6/1
  Demux2/1 -> Sum/2
  Gain Corrector3/1 -> Sum3/1
  Demux1/2 -> Product/1, Sum7/1
  w/1 -> w*Lf_pu/1
  Sum7/1 -> Mux/2  "is_q*"
  Sum3/1 -> Mux/1  "is_d*"
  Sum5/1 -> Gain Corrector2/1
  Sum6/1 -> Sum5/2
  Demux/2 -> Sum6/2
  Mux/1 -> Is_dq*/1
  Sum2/1 -> Gain Corrector3/1
  Product/1 -> Sum2/2
  w*Lf_pu/1 -> Product/2, Product1/1
  Sum/1 -> Sum2/1
  Demux1/1 -> Product1/2, Sum3/2
  Demux/1 -> Sum/1
  Vm_dq*/1 -> Demux/1
  Is_dq/1 -> Demux1/1
  Eg_dq/1 -> Demux2/1

== system GFo_Lib/2-Level LCL-filter/Control loops/Direct AC Voltage control/Current Limitation/Current control ==
  Ig_dq0* : Inport
  Is_dq0 : Inport  Port=2
  vpcc_dq0 : Inport  Port=3
  w : Inport  Port=4
  Demux : Demux  Outputs=2
  Demux1 : Demux  Outputs=2
  Demux2 : Demux  Outputs=2
  Gain Corrector : Gain  Gain=3/(Tr_I_max/1000)*Lf_pu
  Gain Corrector1 : Gain  Gain=3/(Tr_I_max/1000)*Lf_pu
  Mux : Mux  Inputs=2
  Product : Product  RndMeth=Zero
  Product1 : Product  RndMeth=Zero
  Sum : Sum  Inputs=|+-
  Sum2 : Sum  Inputs=|+-
  Sum3 : Sum  Inputs=|++
  Sum5 : Sum  Inputs=++|
  Sum6 : Sum  Inputs=-+|
  Sum7 : Sum  Inputs=++|
  vpcc_abc{1,3..6} (5 alike) : Scope
  w*Lf_pu : Gain  Gain=Lf_pu
  vm : Outport  InitialOutput=0  VectorParamsAs1DForOutWhenUnconnected=off
  wires:
  Mux/1 -> vm/1
  Ig_dq0*/1 -> Demux/1, vpcc_abc4/1
  Sum6/1 -> Gain Corrector1/1
  vpcc_dq0/1 -> vpcc_abc6/1, Demux2/1
  Is_dq0/1 -> Demux1/1
  Demux/1 -> Sum/1
  Demux1/1 -> Product1/2, Sum/2
  Gain Corrector/1 -> Sum2/1
  w*Lf_pu/1 -> Product1/1, Product/2
  Demux1/2 -> Product/1, Sum6/1
  Product/1 -> Sum2/2
  Sum2/1 -> Sum3/1
  Demux/2 -> Sum6/2
  Gain Corrector1/1 -> Sum5/2
  Product1/1 -> Sum5/1
  Sum5/1 -> Sum7/2
  Sum3/1 -> vpcc_abc3/1, Mux/1  "Vm_d*"
  Sum7/1 -> Mux/2  "Vm_q*"
  Sum/1 -> Gain Corrector/1, vpcc_abc1/1
  w/1 -> w*Lf_pu/1, vpcc_abc5/1
  Demux2/1 -> Sum3/2
  Demux2/2 -> Sum7/1

== system GFo_Lib/2-Level LCL-filter/Control loops/Direct AC Voltage control/Current Limitation/Inverse Current control ==
  Vm_dq* : Inport
  Is_dq : Inport  Port=2
  Eg_dq : Inport  Port=3
  w : Inport  Port=4
  Demux : Demux  Outputs=2
  Demux1 : Demux  Outputs=2
  Demux2 : Demux  Outputs=2
  Gain Corrector2 : Gain  Gain=1/(3/(Tr_I_max/1000)*Lf_pu)
  Gain Corrector3 : Gain  Gain=1/(3/(Tr_I_max/1000)*Lf_pu)
  Mux : Mux  Inputs=2
  Product : Product  RndMeth=Zero
  Product1 : Product  RndMeth=Zero
  Sum : Sum  Inputs=|+-
  Sum2 : Sum  Inputs=|++
  Sum3 : Sum  Inputs=|++
  Sum5 : Sum  Inputs=-+|
  Sum6 : Sum  Inputs=-+|
  Sum7 : Sum  Inputs=++|
  w*Lf_pu : Gain  Gain=Lf_pu
  Is_dq* : Outport  InitialOutput=0  VectorParamsAs1DForOutWhenUnconnected=off
  wires:
  Gain Corrector2/1 -> Sum7/2
  Product1/1 -> Sum5/1
  Demux2/2 -> Sum6/1
  Demux2/1 -> Sum/2
  Gain Corrector3/1 -> Sum3/1
  Demux1/2 -> Product/1, Sum7/1
  w/1 -> w*Lf_pu/1
  Sum7/1 -> Mux/2  "is_q*"
  Sum3/1 -> Mux/1  "is_d*"
  Sum5/1 -> Gain Corrector2/1
  Sum6/1 -> Sum5/2
  Demux/2 -> Sum6/2
  Mux/1 -> Is_dq*/1
  Sum2/1 -> Gain Corrector3/1
  Product/1 -> Sum2/2
  w*Lf_pu/1 -> Product/2, Product1/1
  Sum/1 -> Sum2/1
  Demux1/1 -> Product1/2, Sum3/2
  Demux/1 -> Sum/1
  Vm_dq*/1 -> Demux/1
  Is_dq/1 -> Demux1/1
  Eg_dq/1 -> Demux2/1
